simulink model "Model"  (R2023a)
settings: Solver=FixedStepAuto  StartTime=0.0  StopTime=200  FixedStep=0.0001  RelTol=1e-3
values from neighbouring files (symbols this model uses):
  Ac = [0      1       0           0 ... (first row only)    [MS_PID.m]    (also in MS_PID2020a.m)
  amp = 0.0005    [MS_PID.m]    (also in MS_PID2020a.m = 0.0001)
  An = [0 1 ... (first row only)    [MS_PID.m]    (also in MS_PID2020a.m)
  Bc = [0 +k_f/m 0 -k_f/M]'    [MS_PID.m]    (also in MS_PID2020a.m)
  Bn = [0 0]'    [MS_PID.m]    (also in MS_PID2020a.m)
  Cc = [-k_m/m -c_m/m   k_m/m       c_m/m ... (first row only)    [MS_PID.m]    (also in MS_PID2020a.m)
  Cn = [1 0]    [MS_PID.m]    (also in MS_PID2020a.m)
  Dc = [+k_f/m -k_f/M]'    [MS_PID.m]    (also in MS_PID2020a.m)
  den = [L R_m]    [MS_PID.m]    (also in MS_PID2020a.m)
  Dn = 0    [MS_PID.m]    (also in MS_PID2020a.m)
  Ec = [0 0 0 c_M/M ... (first row only)    [MS_PID.m]    (also in MS_PID2020a.m)
  En = [0 0 ... (first row only)    [MS_PID.m]    (also in MS_PID2020a.m)
  fre = 45    [MS_PID.m]    (also in MS_PID2020a.m)
  k_E = 0    [MS_PID.m]    (also in MS_PID2020a.m)
  Kd = 00070    (= 70)    [MS_PID.m]    (also in MS_PID2020a.m)
  Ki = 13000    [MS_PID.m]    (also in MS_PID2020a.m)
  Kp = 27000    [MS_PID.m]    (also in MS_PID2020a.m)
  num = 1    [MS_PID.m]    (also in MS_PID2020a.m)
libraries: slpidlib x3
settings Model: Creator=z'k'x  LastModifiedBy=z'k'x

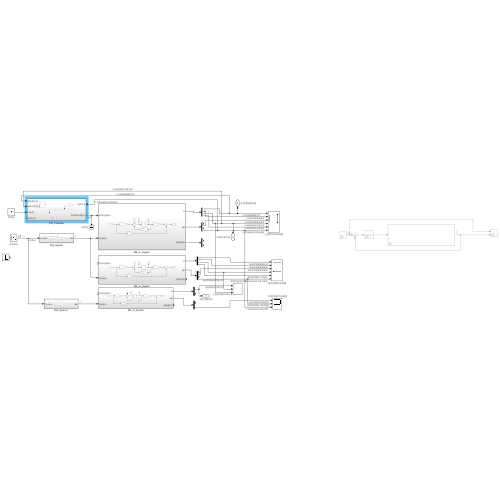
[thumbnail: Simulink's stored preview of the top-level diagram]
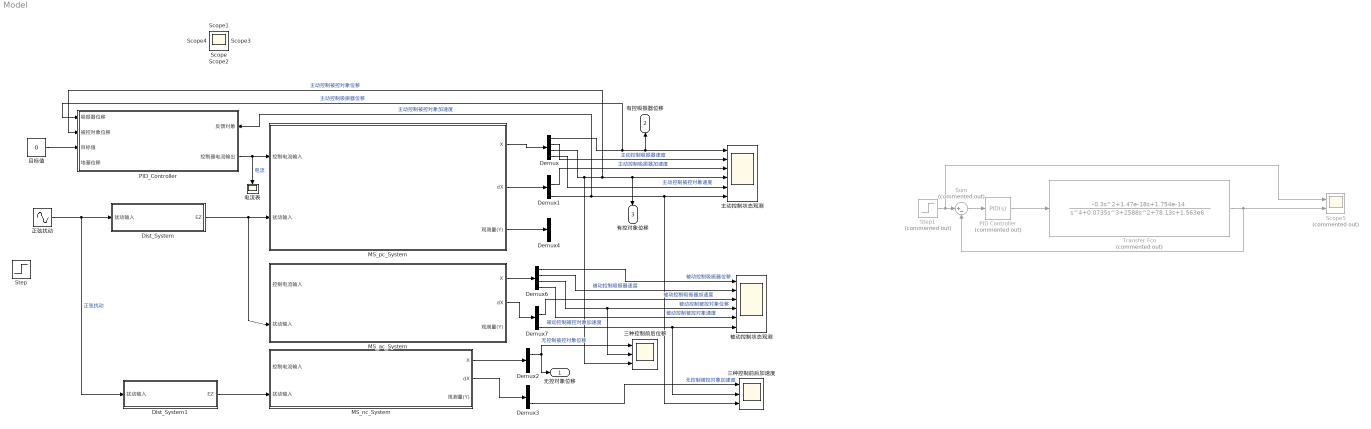
== system Model ==
  Demux{,1,6..7} (4 alike) : Demux
  Demux2 : Demux  Outputs=2
  Demux3 : Demux  Outputs=2
  Demux4 : Demux  Outputs=2
  Dist_System : Subsystem
  Dist_System1 : Subsystem
  MS_ac_System : Subsystem
  MS_nc_System : Subsystem
  MS_pc_System : Subsystem
  PID Controller : slpidlib/PID Controller  Commented=on  Controller=PID  Form=Parallel  TimeDomain=Continuous-time  UseExternalTs=off  SampleTime=-1  IntegratorMethod=Forward Euler  FilterMethod=Forward Euler  ControllerParametersSource=internal  P=100  I=100  UseKiTs=off  D=0  N=100  UseFilter=on  TunerSelectOption=Transfer Function Based (PID Tuner App)  InitialConditionSource=internal  InitialConditionForIntegrator=0  InitialConditionForFilter=0  DifferentiatorICPrevScaledInput=0  ExternalReset=none  TrackingMode=off  Kt=1  LimitOutput=off  SatLimitsSource=internal  UpperSaturationLimit=inf  LowerSaturationLimit=-inf  LinearizeAsGain=on  AntiWindupMode=none  Kb=1  LimitIntegrator=off  UpperIntegratorSaturationLimit=inf  LowerIntegratorSaturationLimit=-inf  POutMin=[]  POutMax=[]  IOutMin=[]  IOutMax=[]  DOutMin=[]  DOutMax=[]  NOutMin=[]  NOutMax=[]  SumOutMin=[]  SumOutMax=[]  SaturationOutMin=[]  SaturationOutMax=[]  PParamMin=[]  PParamMax=[]  IParamMin=[]  IParamMax=[]  DParamMin=[]  DParamMax=[]  NParamMin=[]  NParamMax=[]  KbParamMin=[]  KbParamMax=[]  KtParamMin=[]  KtParamMax=[]  KbOutMin=[]  KbOutMax=[]  KtOutMin=[]  KtOutMax=[]  IntegratorOutMin=[]  IntegratorOutMax=[]  FilterOutMin=[]  FilterOutMax=[]  SumI1OutMin=[]  SumI1OutMax=[]  SumI2OutMin=[]  SumI2OutMax=[]  SumI3OutMin=[]  SumI3OutMax=[]  SumI4OutMin=[]  SumI4OutMax=[]  SumDOutMin=[]  SumDOutMax=[]  DifferentiatorOutMin=[]  DifferentiatorOutMax=[]  FilterDiffOutCoefMin=[]  FilterDiffOutCoefMax=[]  ReciprocalOutMin=[]  ReciprocalOutMax=[]  SumDenOutMin=[]  SumDenOutMax=[]  SumNumOutMin=[]  SumNumOutMax=[]  DivideOutMin=[]  DivideOutMax=[]  UdiffTsProdOutMin=[]  UdiffTsProdOutMax=[]  NTsProdOutMin=[]  NTsProdOutMax=[]  UintegralTsProdOutMin=[]  UintegralTsProdOutMax=[]  UngainTsProdOutMin=[]  UngainTsProdOutMax=[]  ClampingZeroOutDataTypeStr=Inherit: Inherit via back propagation  ClampingZeroOutMin=[]  ClampingZeroOutMax=[]  FilterDenConstantOutDataTypeStr=Inherit: Inherit via back propagation  FilterDenConstantOutMin=[]  FilterDenConstantOutMax=[]  PCopyOutDataTypeStr=Inherit: Inherit via back propagation  PCopyOutMin=[]  PCopyOutMax=[]  NCopyOutDataTypeStr=Inherit: Inherit via back propagation  NCopyOutMin=[]  NCopyOutMax=[]  IntegratorContinuousStateAttributes=''  IntegratorStateMustResolveToSignalObject=off  IntegratorRTWStateStorageClass=Auto  FilterContinuousStateAttributes=''  FilterStateMustResolveToSignalObject=off  FilterRTWStateStorageClass=Auto  ParallelPVariant=InternalParameters  IdealPVariant=Disabled  IVariant=InternalParameters  DVariant=InternalParameters  IntegratorVariant=Continuous  SatVariant=Disabled  AWVariant=Passthrough  PCopyVariant=Disabled  TRVariant=Disabled  FdbkBlocksVariant=Forward  IdealPFdbkVariant=Disabled  SatFdbkVariant=Disabled  DerivativeFilterVariant=ContFilter  NVariant=InternalParameters  NCopyVariant=Disabled  FilterICVariant=InternalICsFilter  IntegratorICVariant=InternalICs  ExternalResetVariant=Disabled  TRSumVariant=Passthrough  SumFdbkVariant=Disabled  SumVariant=Sum_PID  TsampFilterVariant=InternalTs  TsampNgainVariant=Passthrough  TsampIntegralVariant=Disabled_SignalSpec  ExternalSaturationOutDataTypeStr=Inherit: Same as second input
  PID_Controller : Subsystem
      settings: PortSchema="{\"entries\":[{\"content\":{\"sides\":[{\"content\":{\"connectorIds\":[\"In1\",\"In2\",\"In3\",\"In4\"]},\"type\":\"ConnectorPlacement.EquallySpacedRectSide\",\"uuid\":\"571e86c5-cb6d-479a-9436-f1f62a1aff4a\"},{\"content\":{\"connectorIds\":[\"In5\",\"Out1\"],\"side\":\"RIGHT\"},\"type\":\"ConnectorPlacement.EquallySpacedRectSide\",\"uuid\":\"8a3b2c99-baa4-4442-bf6b-a8e33bce6e66\"},{\"content\":{\"side\":\"TOP\"},\"type\":\"ConnectorPlacement.EquallySpacedRectSide\",\"uuid\":\"097c69f3-d0cb-436f-a6ca-a824d158c0f7\"}]},\"type\":\"ConnectorPlacement.EquallySpacedConnector\",\"uuid\":\"d0159daf-3351-4c39-bc94-0e104d76ad45\"}],\"packageUris\":[\"http://schema.mathworks.com/mf0/Connector/R2020b\"],\"version\":\"1.0\"}"
  Scope5 : Scope  Commented=on  NumInputPorts=2
  Step : Step  Before=0.002  After=0  SampleTime=0
  Step1 : Step  Commented=on  After=0.00001  SampleTime=0
  Sum : Sum  Commented=on  Inputs=|+-
  Transfer Fcn : TransferFcn  Commented=on  Numerator=[-0.3 1.47e-18 1.754e-14]  Denominator=[1 0.0735 2588 78.13 1.563e6]
  三种控制前后位移 : Scope  NumInputPorts=3
  三种控制前后加速度 : Scope  NumInputPorts=3
  主动控制状态观测 : Scope  NumInputPorts=6
  正弦扰动 : Sin  Amplitude=amp  Frequency=fre  SampleTime=0
  电流表 : Scope
  目标值 : Constant  Value=0
  被动控制状态观测 : Scope  NumInputPorts=6
  无控对象位移 : Outport
  有控吸振器位移 : Outport  Port=2
  有控对象位移 : Outport  Port=3
  Scope{,1..4} (5 alike) : Scope
  wires:
  MS_pc_System/1(X) -> Demux/1
  MS_pc_System/2(dX) -> Demux1/1
  Demux/1 -> 主动控制状态观测/1, 有控吸振器位移/1, PID_Controller/1(吸振器位移)  "主动控制吸振器位移"
  Demux/2 -> 主动控制状态观测/2  "主动控制吸振器速度"
  Demux1/2 -> 主动控制状态观测/3  "主动控制吸振器加速度"
  Demux1/4 -> 主动控制状态观测/6, 三种控制前后加速度/3, PID_Controller/5(反馈对象)  "主动控制被控对象加速度"
  Demux/3 -> 三种控制前后位移/3, PID_Controller/2(被控对象位移), 主动控制状态观测/4, 有控对象位移/1  "主动控制被控对象位移"
  Demux/4 -> 主动控制状态观测/5  "主动控制被控对象速度"
  正弦扰动/1 -> Dist_System1/1(扰动输入), Dist_System/1(扰动输入)  "正弦扰动"
  Demux2/1 -> 无控对象位移/1, 三种控制前后位移/1  "无控制被控对象位移"
  PID_Controller/1(控制器电流输出) -> 电流表/1, MS_pc_System/1(控制电流输入)  "电流"
  Demux3/2 -> 三种控制前后加速度/1  "无控制被控对象加速度"
  目标值/1 -> PID_Controller/3(目标值)
  PID Controller/1 -> Transfer Fcn/1
  Step1/1 -> Scope5/1, Sum/1
  Transfer Fcn/1 -> Sum/2, Scope5/2
  Sum/1 -> PID Controller/1
  MS_nc_System/1(X) -> Demux2/1
  MS_nc_System/2(dX) -> Demux3/1
  Dist_System/1(EZ) -> MS_ac_System/2(扰动输入), MS_pc_System/2(扰动输入)
  Demux7/4 -> 三种控制前后加速度/2, 被动控制状态观测/6  "被动控制被控对象加速度"
  Demux6/1 -> 被动控制状态观测/1  "被动控制吸振器位移"
  MS_ac_System/2(dX) -> Demux7/1
  Demux6/3 -> 三种控制前后位移/2, 被动控制状态观测/4  "被动控制被控对象位移"
  MS_ac_System/1(X) -> Demux6/1
  Demux7/2 -> 被动控制状态观测/3  "被动控制吸振器加速度"
  Demux6/4 -> 被动控制状态观测/5  "被动控制被控对象速度"
  Demux6/2 -> 被动控制状态观测/2  "被动控制吸振器速度"
  MS_pc_System/3(观测量(Y)) -> Demux4/1
  Dist_System1/1(EZ) -> MS_nc_System/2(扰动输入)

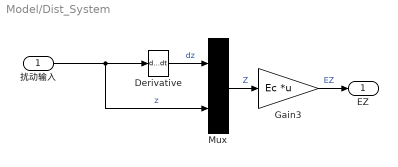
== system Model/Dist_System ==
  扰动输入 : Inport
  Derivative : Derivative
  Gain3 : Gain  Gain=Ec  Multiplication=Matrix(K*u) (u vector)
  Mux : Mux  Inputs=2
      settings: DisplayOption=signals
  EZ : Outport
  wires:
  Gain3/1 -> EZ/1  "EZ"
  Mux/1 -> Gain3/1  "Z"
  Derivative/1 -> Mux/1  "dz"
  扰动输入/1 -> Derivative/1, Mux/2  "z"

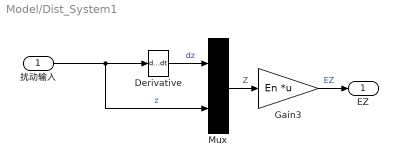
== system Model/Dist_System1 ==
  扰动输入 : Inport
  Derivative : Derivative
  Gain3 : Gain  Gain=En  Multiplication=Matrix(K*u) (u vector)
  Mux : Mux  Inputs=2
      settings: DisplayOption=signals
  EZ : Outport
  wires:
  Gain3/1 -> EZ/1  "EZ"
  Mux/1 -> Gain3/1  "Z"
  Derivative/1 -> Mux/1  "dz"
  扰动输入/1 -> Derivative/1, Mux/2  "z"

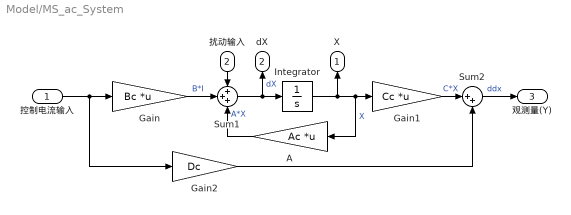
== system Model/MS_ac_System ==
  控制电流输入 : Inport
  扰动输入 : Inport  Port=2
  A : Gain  Gain=Ac  Multiplication=Matrix(K*u) (u vector)
  Gain : Gain  Gain=Bc  Multiplication=Matrix(K*u) (u vector)
  Gain1 : Gain  Gain=Cc  Multiplication=Matrix(K*u) (u vector)
  Gain2 : Gain  Gain=Dc
  Integrator : Integrator
  Sum1 : Sum  Inputs=+++
  Sum2 : Sum  Inputs=|++
  X : Outport
  dX : Outport  Port=2
  观测量(Y) : Outport  Port=3
  wires:
  扰动输入/1 -> Sum1/1
  控制电流输入/1 -> Gain2/1, Gain/1
  Sum2/1 -> 观测量(Y)/1  "ddx"
  A/1 -> Sum1/3  "A*X"
  Gain1/1 -> Sum2/1  "C*X"
  Gain/1 -> Sum1/2  "B*I"
  Sum1/1 -> Integrator/1, dX/1  "dX"
  Integrator/1 -> X/1, A/1, Gain1/1  "X"
  Gain2/1 -> Sum2/2

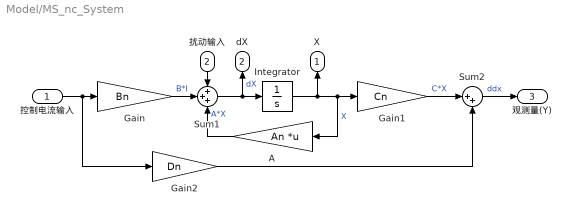
== system Model/MS_nc_System ==
  控制电流输入 : Inport
  扰动输入 : Inport  Port=2
  A : Gain  Gain=An  Multiplication=Matrix(K*u) (u vector)
  Gain : Gain  Gain=Bn
  Gain1 : Gain  Gain=Cn
  Gain2 : Gain  Gain=Dn
  Integrator : Integrator
  Sum1 : Sum  Inputs=+++
  Sum2 : Sum  Inputs=|++
  X : Outport
  dX : Outport  Port=2
  观测量(Y) : Outport  Port=3
  wires:
  Gain2/1 -> Sum2/2
  Integrator/1 -> A/1, Gain1/1, X/1  "X"
  Sum1/1 -> dX/1, Integrator/1  "dX"
  Gain/1 -> Sum1/2  "B*I"
  Gain1/1 -> Sum2/1  "C*X"
  A/1 -> Sum1/3  "A*X"
  Sum2/1 -> 观测量(Y)/1  "ddx"
  控制电流输入/1 -> Gain/1, Gain2/1
  扰动输入/1 -> Sum1/1

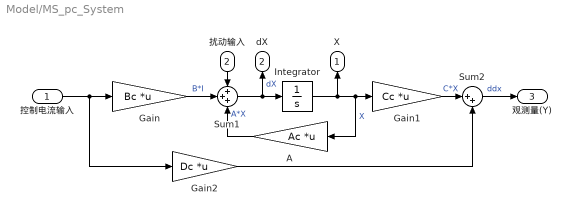
== system Model/MS_pc_System ==
  控制电流输入 : Inport
  扰动输入 : Inport  Port=2
  A : Gain  Gain=Ac  Multiplication=Matrix(K*u) (u vector)
  Gain : Gain  Gain=Bc  Multiplication=Matrix(K*u) (u vector)
  Gain1 : Gain  Gain=Cc  Multiplication=Matrix(K*u) (u vector)
  Gain2 : Gain  Gain=Dc  Multiplication=Matrix(K*u) (u vector)
  Integrator : Integrator
  Sum1 : Sum  Inputs=+++
  Sum2 : Sum  Inputs=|++
  X : Outport
  dX : Outport  Port=2
  观测量(Y) : Outport  Port=3
  wires:
  Gain2/1 -> Sum2/2
  Integrator/1 -> Gain1/1, A/1, X/1  "X"
  Sum1/1 -> dX/1, Integrator/1  "dX"
  Gain/1 -> Sum1/2  "B*I"
  Gain1/1 -> Sum2/1  "C*X"
  A/1 -> Sum1/3  "A*X"
  Sum2/1 -> 观测量(Y)/1  "ddx"
  控制电流输入/1 -> Gain/1, Gain2/1
  扰动输入/1 -> Sum1/1

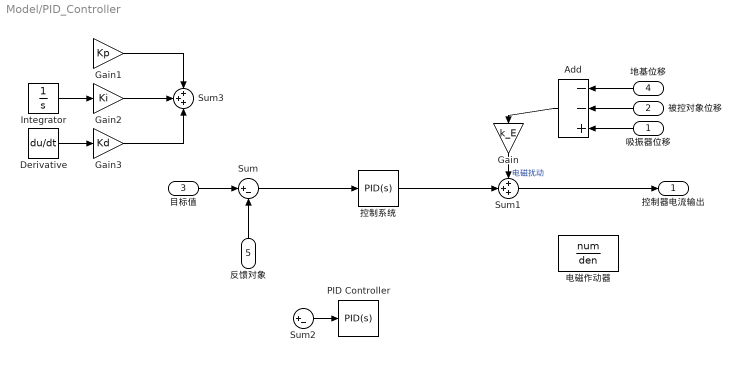
== system Model/PID_Controller ==
  吸振器位移 : Inport
  被控对象位移 : Inport  Port=2
  目标值 : Inport  Port=3
  地基位移 : Inport  Port=4
  反馈对象 : Inport  Port=5
  Add : Sum  Inputs=--+
  Derivative : Derivative
  Gain : Gain  Gain=k_E
  Gain1 : Gain  Gain=Kp
  Gain2 : Gain  Gain=Ki
  Gain3 : Gain  Gain=Kd
  Integrator : Integrator
  PID Controller : slpidlib/PID Controller  Controller=PID  Form=Parallel  TimeDomain=Continuous-time  UseExternalTs=off  SampleTime=-1  IntegratorMethod=Forward Euler  FilterMethod=Forward Euler  ControllerParametersSource=internal  P=1200  I=700  UseKiTs=off  D=-0.1  N=100  UseFilter=on  TunerSelectOption=Transfer Function Based (PID Tuner App)  InitialConditionSource=internal  InitialConditionForIntegrator=0  InitialConditionForFilter=0  DifferentiatorICPrevScaledInput=0  ExternalReset=none  TrackingMode=off  Kt=1  LimitOutput=off  SatLimitsSource=internal  UpperSaturationLimit=inf  LowerSaturationLimit=-inf  LinearizeAsGain=on  AntiWindupMode=none  Kb=1  LimitIntegrator=off  UpperIntegratorSaturationLimit=inf  LowerIntegratorSaturationLimit=-inf  POutMin=[]  POutMax=[]  IOutMin=[]  IOutMax=[]  DOutMin=[]  DOutMax=[]  NOutMin=[]  NOutMax=[]  SumOutMin=[]  SumOutMax=[]  SaturationOutMin=[]  SaturationOutMax=[]  PParamMin=[]  PParamMax=[]  IParamMin=[]  IParamMax=[]  DParamMin=[]  DParamMax=[]  NParamMin=[]  NParamMax=[]  KbParamMin=[]  KbParamMax=[]  KtParamMin=[]  KtParamMax=[]  KbOutMin=[]  KbOutMax=[]  KtOutMin=[]  KtOutMax=[]  IntegratorOutMin=[]  IntegratorOutMax=[]  FilterOutMin=[]  FilterOutMax=[]  SumI1OutMin=[]  SumI1OutMax=[]  SumI2OutMin=[]  SumI2OutMax=[]  SumI3OutMin=[]  SumI3OutMax=[]  SumI4OutMin=[]  SumI4OutMax=[]  SumDOutMin=[]  SumDOutMax=[]  DifferentiatorOutMin=[]  DifferentiatorOutMax=[]  FilterDiffOutCoefMin=[]  FilterDiffOutCoefMax=[]  ReciprocalOutMin=[]  ReciprocalOutMax=[]  SumDenOutMin=[]  SumDenOutMax=[]  SumNumOutMin=[]  SumNumOutMax=[]  DivideOutMin=[]  DivideOutMax=[]  UdiffTsProdOutMin=[]  UdiffTsProdOutMax=[]  NTsProdOutMin=[]  NTsProdOutMax=[]  UintegralTsProdOutMin=[]  UintegralTsProdOutMax=[]  UngainTsProdOutMin=[]  UngainTsProdOutMax=[]  ClampingZeroOutDataTypeStr=Inherit: Inherit via back propagation  ClampingZeroOutMin=[]  ClampingZeroOutMax=[]  FilterDenConstantOutDataTypeStr=Inherit: Inherit via back propagation  FilterDenConstantOutMin=[]  FilterDenConstantOutMax=[]  PCopyOutDataTypeStr=Inherit: Inherit via back propagation  PCopyOutMin=[]  PCopyOutMax=[]  NCopyOutDataTypeStr=Inherit: Inherit via back propagation  NCopyOutMin=[]  NCopyOutMax=[]  IntegratorContinuousStateAttributes=''  IntegratorStateMustResolveToSignalObject=off  IntegratorRTWStateStorageClass=Auto  FilterContinuousStateAttributes=''  FilterStateMustResolveToSignalObject=off  FilterRTWStateStorageClass=Auto  ParallelPVariant=InternalParameters  IdealPVariant=Disabled  IVariant=InternalParameters  DVariant=InternalParameters  IntegratorVariant=Continuous  SatVariant=Disabled  AWVariant=Passthrough  PCopyVariant=Disabled  TRVariant=Disabled  FdbkBlocksVariant=Forward  IdealPFdbkVariant=Disabled  SatFdbkVariant=Disabled  DerivativeFilterVariant=ContFilter  NVariant=InternalParameters  NCopyVariant=Disabled  FilterICVariant=InternalICsFilter  IntegratorICVariant=InternalICs  ExternalResetVariant=Disabled  TRSumVariant=Passthrough  SumFdbkVariant=Disabled  SumVariant=Sum_PID  TsampFilterVariant=InternalTs  TsampNgainVariant=Passthrough  TsampIntegralVariant=Disabled_SignalSpec  ExternalSaturationOutDataTypeStr=Inherit: Same as second input
  Sum : Sum  Inputs=|+-
  Sum1 : Sum  Inputs=+++
  Sum2 : Sum  Inputs=|+-
  Sum3 : Sum  Inputs=+++
  控制系统 : slpidlib/PID Controller  Controller=PID  Form=Parallel  TimeDomain=Continuous-time  UseExternalTs=off  SampleTime=-1  IntegratorMethod=Forward Euler  FilterMethod=Forward Euler  ControllerParametersSource=internal  P=Kp  I=Ki  UseKiTs=off  D=Kd  N=100  UseFilter=on  TunerSelectOption=Transfer Function Based (PID Tuner App)  InitialConditionSource=internal  InitialConditionForIntegrator=0  InitialConditionForFilter=0  DifferentiatorICPrevScaledInput=0  ExternalReset=none  TrackingMode=off  Kt=1  LimitOutput=off  SatLimitsSource=internal  UpperSaturationLimit=inf  LowerSaturationLimit=-inf  LinearizeAsGain=on  AntiWindupMode=none  Kb=1  LimitIntegrator=off  UpperIntegratorSaturationLimit=inf  LowerIntegratorSaturationLimit=-inf  POutMin=[]  POutMax=[]  IOutMin=[]  IOutMax=[]  DOutMin=[]  DOutMax=[]  NOutMin=[]  NOutMax=[]  SumOutMin=[]  SumOutMax=[]  SaturationOutMin=[]  SaturationOutMax=[]  PParamMin=[]  PParamMax=[]  IParamMin=[]  IParamMax=[]  DParamMin=[]  DParamMax=[]  NParamMin=[]  NParamMax=[]  KbParamMin=[]  KbParamMax=[]  KtParamMin=[]  KtParamMax=[]  KbOutMin=[]  KbOutMax=[]  KtOutMin=[]  KtOutMax=[]  IntegratorOutMin=[]  IntegratorOutMax=[]  FilterOutMin=[]  FilterOutMax=[]  SumI1OutMin=[]  SumI1OutMax=[]  SumI2OutMin=[]  SumI2OutMax=[]  SumI3OutMin=[]  SumI3OutMax=[]  SumI4OutMin=[]  SumI4OutMax=[]  SumDOutMin=[]  SumDOutMax=[]  DifferentiatorOutMin=[]  DifferentiatorOutMax=[]  FilterDiffOutCoefMin=[]  FilterDiffOutCoefMax=[]  ReciprocalOutMin=[]  ReciprocalOutMax=[]  SumDenOutMin=[]  SumDenOutMax=[]  SumNumOutMin=[]  SumNumOutMax=[]  DivideOutMin=[]  DivideOutMax=[]  UdiffTsProdOutMin=[]  UdiffTsProdOutMax=[]  NTsProdOutMin=[]  NTsProdOutMax=[]  UintegralTsProdOutMin=[]  UintegralTsProdOutMax=[]  UngainTsProdOutMin=[]  UngainTsProdOutMax=[]  ClampingZeroOutDataTypeStr=Inherit: Inherit via back propagation  ClampingZeroOutMin=[]  ClampingZeroOutMax=[]  FilterDenConstantOutDataTypeStr=Inherit: Inherit via back propagation  FilterDenConstantOutMin=[]  FilterDenConstantOutMax=[]  PCopyOutDataTypeStr=Inherit: Inherit via back propagation  PCopyOutMin=[]  PCopyOutMax=[]  NCopyOutDataTypeStr=Inherit: Inherit via back propagation  NCopyOutMin=[]  NCopyOutMax=[]  IntegratorContinuousStateAttributes=''  IntegratorStateMustResolveToSignalObject=off  IntegratorRTWStateStorageClass=Auto  FilterContinuousStateAttributes=''  FilterStateMustResolveToSignalObject=off  FilterRTWStateStorageClass=Auto  ParallelPVariant=InternalParameters  IdealPVariant=Disabled  IVariant=InternalParameters  DVariant=InternalParameters  IntegratorVariant=Continuous  SatVariant=Disabled  AWVariant=Passthrough  PCopyVariant=Disabled  TRVariant=Disabled  FdbkBlocksVariant=Forward  IdealPFdbkVariant=Disabled  SatFdbkVariant=Disabled  DerivativeFilterVariant=ContFilter  NVariant=InternalParameters  NCopyVariant=Disabled  FilterICVariant=InternalICsFilter  IntegratorICVariant=InternalICs  ExternalResetVariant=Disabled  TRSumVariant=Passthrough  SumFdbkVariant=Disabled  SumVariant=Sum_PID  TsampFilterVariant=InternalTs  TsampNgainVariant=Passthrough  TsampIntegralVariant=Disabled_SignalSpec  ExternalSaturationOutDataTypeStr=Inherit: Same as second input
  电磁作动器 : TransferFcn  Numerator=num  Denominator=den
  控制器电流输出 : Outport
  wires:
  Add/1 -> Gain/1
  反馈对象/1 -> Sum/2
  地基位移/1 -> Add/1
  Gain/1 -> Sum1/1  "电磁扰动"
  吸振器位移/1 -> Add/3
  目标值/1 -> Sum/1
  被控对象位移/1 -> Add/2
  控制系统/1 -> Sum1/2
  Sum/1 -> 控制系统/1
  Sum2/1 -> PID Controller/1
  ? -> Derivative/1
  ? -> Integrator/1
  Derivative/1 -> Gain3/1
  Gain2/1 -> Sum3/2
  Gain1/1 -> Sum3/1
  ? -> Gain1/1
  Gain3/1 -> Sum3/3
  Integrator/1 -> Gain2/1
  Sum1/1 -> 控制器电流输出/1
